simulink model "EngineControl_Overview"  (R2018a)
settings: Solver=VariableStepAuto  StartTime=0.0  StopTime=20  MaxStep=0.01  RelTol=1e-9
settings Model: Creator=rahul  LastModifiedBy=rahul

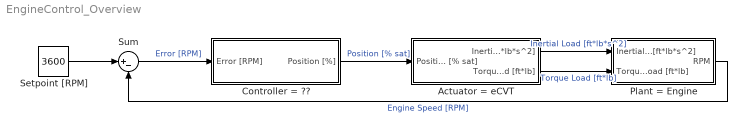
== system EngineControl_Overview ==
  Actuator = eCVT : Subsystem
  Controller = ?? : Subsystem
  Plant = Engine : Subsystem
  Setpoint [RPM] : Constant  Value=3600
  Sum : Sum  Inputs=|+-
  wires:
  Setpoint [RPM]/1 -> Sum/1
  Sum/1 -> Controller = ??/1(Error [RPM])  "Error [RPM]"
  Actuator = eCVT/1(Inertial Load [ft*lb*s^2]) -> Plant = Engine/1(Inertial Load [ft*lb*s^2])  "Inertial Load [ft*lb*s^2]"
  Controller = ??/1(Position [%]) -> Actuator = eCVT/1(Position [% sat])  "Position [% sat]"
  Actuator = eCVT/2(Torque Load [ft*lb]) -> Plant = Engine/2(Torque Load [ft*lb])  "Torque Load [ft*lb]"
  Plant = Engine/1(RPM) -> Sum/2  "Engine Speed [RPM]"

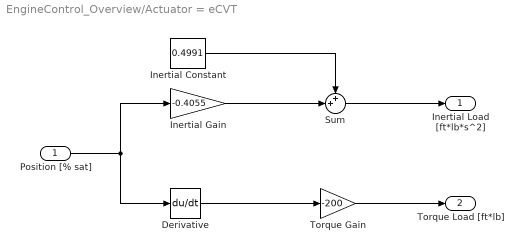
== system EngineControl_Overview/Actuator = eCVT ==
  Position [% sat] : Inport
  "Derivative " : Derivative
  Inertial Constant : Constant  Value=0.4991
  Inertial Gain : Gain  Gain=-0.4055
  Sum : Sum  Inputs=++|
  Torque Gain : Gain  Gain=-200
  Inertial Load [ft*lb*s^2] : Outport
  Torque Load [ft*lb] : Outport  Port=2
  wires:
  Position [% sat]/1 -> Inertial Gain/1, "Derivative "/1
  Sum/1 -> Inertial Load [ft*lb*s^2]/1
  Inertial Gain/1 -> Sum/2
  Inertial Constant/1 -> Sum/1
  "Derivative "/1 -> Torque Gain/1
  Torque Gain/1 -> Torque Load [ft*lb]/1

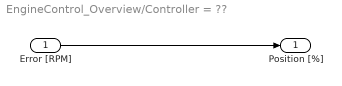
== system EngineControl_Overview/Controller = ?? ==
  Error [RPM] : Inport
  Position [%] : Outport
  wires:
  Error [RPM]/1 -> Position [%]/1

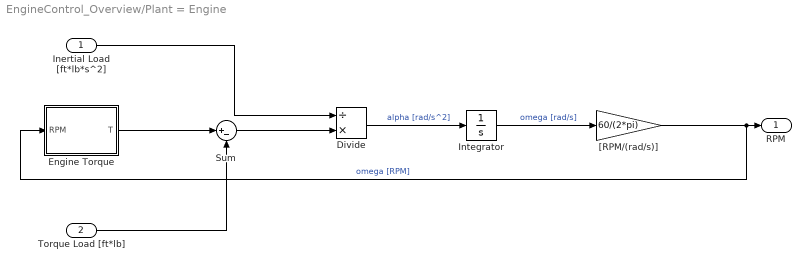
== system EngineControl_Overview/Plant = Engine ==
  Inertial Load [ft*lb*s^2] : Inport
  Torque Load [ft*lb] : Inport  Port=2
  Divide : Product  Inputs=/*
  Engine Torque : MATLAB Function  TreatAsAtomicUnit=on
  "Integrator " : Integrator  InitialCondition=3000*(2*pi)/60
  Sum : Sum  Inputs=|+-
  "[RPM/(rad/s)]" : Gain  Gain=60/(2*pi)
  RPM : Outport
  wires:
  "Integrator "/1 -> "[RPM/(rad/s)]"/1  "omega [rad/s]"
  "[RPM/(rad/s)]"/1 -> Engine Torque/1(RPM), RPM/1  "omega [RPM]"
  Divide/1 -> "Integrator "/1  "alpha [rad/s^2]"
  Engine Torque/1(T) -> Sum/1
  Torque Load [ft*lb]/1 -> Sum/2
  Sum/1 -> Divide/2
  Inertial Load [ft*lb*s^2]/1 -> Divide/1

== matlab function EngineControl_Overview/Plant = Engine/Engine Torque ==
  data: RPM input; T output
function T = fcn(RPM)

% RPM < 1750
if RPM < 1750
    T = 0;

% 1750 < RPM < 3800
elseif RPM < 3600
    % BSM19 Engine HP vs. RPM Equation  (3rd Order)
    HP = - 2.874 * 10^-10 * RPM.^3 ...
         + 1.781 * 10^-06 * RPM.^2 ...
         - 6.842 * 10^-04 * RPM.^1 ...
         + 1.719 * 10^000 * RPM.^0;

    % Torque = Power / Angular Velocity
    T = HP ./ (RPM*2*pi) * 33000;

% 3600 < RPM < 3800
elseif RPM < 3800
    % Linearized Governor
    T = -0.065 * RPM + 247;

% RPM > 3800
else
    T = 0;

end
